simulink subsystem "pressTransducer_MPa"  (R2025a)
settings: Solver=VariableStepAuto  StartTime=0.0  StopTime=10.0  RelTol=1e-3
libraries: nesl_utility x1, fl_lib x1
settings Model: Creator=novatehnika  LastModifiedBy=novatehnika

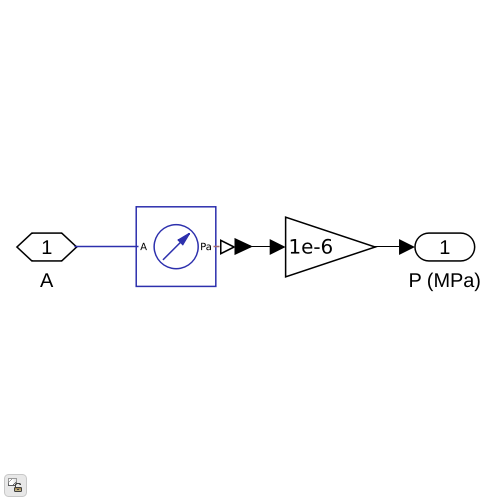
[thumbnail: Simulink's stored preview of the top-level diagram]
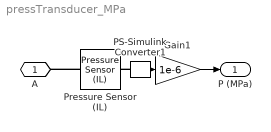
== system pressTransducer_MPa ==
  Gain1 : Gain  Gain=1e-6
  PS-Simulink Converter1 : nesl_utility/PS-Simulink Converter  PhysicalDomain=network_engine_domain  SubClassName=ps_output  LeftPortType=input  RightPortType=output  PseudoPeriodic=off  Frequencies=[]  VectorFormat=1-D array  Unit=Pa  AffineConversion=off
  Pressure Sensor (IL) : fl_lib/Isothermal Liquid/Sensors/Pressure Sensor (IL)  pressure_measure=foundation.enum.pressure_measure.absolute
      settings: InternalSimscapePortConfiguration="{\"Bottom\":[],\"Left\":[{\"id\":\"A\",\"label\":\"A\",\"type\":\"foundation.isothermal_liquid.isothermal_liquid\"}],\"Right\":[{\"id\":\"Pa\",\"label\":\"Pa\",\"type\":\"output\"}],\"Top\":[]}"
  A : PMIOPort  Side=Left
  P (MPa) : Outport
  wires:
  Gain1/1 -> P (MPa)/1
  PS-Simulink Converter1/1 -> Gain1/1
  connections:
  PS-Simulink Converter1/LConn1 -- Pressure Sensor (IL)/RConn1
  Pressure Sensor (IL)/LConn1 -- A/RConn1
